simulink model "kf_continous_time"  (R2018b)
settings: Solver=FixedStepAuto  StartTime=0.0  StopTime=15  FixedStep=1e-3  RelTol=1e-3
undefined symbols (not defined in the file or in its folder): Continuous, Time
libraries: ctrlSharedLib x1, simulink x1
settings Model: Creator=jasprit  LastModifiedBy=jasprit
settings SFSimCC: SimUseLocalCustomCode=off
settings RTWCC: RTWUseLocalCustomCode=off

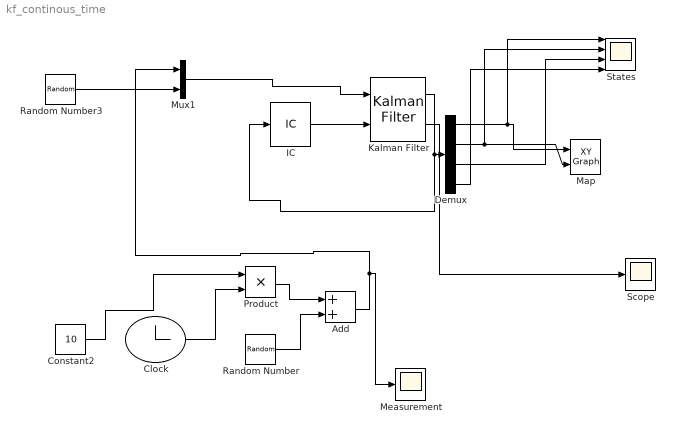
== system kf_continous_time ==
  Add : Sum
  Clock : Clock
  Constant2 : Constant  Value=10
  Demux : Demux
  IC : InitialCondition  Value=[0 0 10 0]
  Kalman Filter : ctrlSharedLib/Kalman Filter  TimeDomain=Continuous-Time  UseCurrentEstimator=on  ModelSource=Individual A, B, C, D matrices  ModelSourceVariable=ss(0.95,1,1,0,1)  A=[0 0 1 0; 0 0 0 1; 0 0 0 0; 0 0 0 0]  B=[1 0; 0 1]  C=[1 0 0 0; 0 1 0 0]  D=[0 0; 0 0]  NumberOfStates=1  NumberOfInputs=1  NumberOfOutputs=1  InitialEstimateSource=Input port  X0=[0 0 20 0]  P0=10  UseK=off  UseGH=off  NumberOfProcessNoiseInputs=1  G=1  TimeInvariantG=on  H=0  TimeInvariantH=on  Q=[0.2 0 0 0; 0 0.2 0 0; 0 0 0.4 0; 0 0 0 0.4]  TimeInvariantQ=on  R=[0.1 0; 0 0.1]  TimeInvariantR=on  N=0  TimeInvariantN=on  AddInputPort=off  AddEnablePort=off  OutputEstimatedY=off  OutputP=on  Ts=-1
      settings: SourceProductBaseCode=CT
  Map : simulink/Sinks/XY Graph  xmin=-1  xmax=200  ymin=-1  ymax=1  st=-1
  "Measurement " : Scope
  Mux1 : Mux  Inputs=2
  Product : Product
  Random Number : RandomNumber  Variance=0.1  SampleTime=0.1
  Random Number3 : RandomNumber  Variance=0.1  SampleTime=0.1
  Scope : Scope
  States : Scope  NumInputPorts=4
  wires:
  Constant2/1 -> Product/1
  Kalman Filter/1 -> Demux/1, IC/1
  Demux/1 -> States/1, Map/1
  Clock/1 -> Product/2
  Product/1 -> Add/1
  Random Number/1 -> Add/2
  Add/1 -> Mux1/1, "Measurement "/1
  Kalman Filter/2 -> Scope/1
  Demux/2 -> Map/2, States/2
  Mux1/1 -> Kalman Filter/1
  Random Number3/1 -> Mux1/2
  Demux/3 -> States/3
  Demux/4 -> States/4
  IC/1 -> Kalman Filter/2
